simulink model "pitch_control_fuzzy"  (R2021b)
settings: Solver=VariableStepAuto  StartTime=0.0  StopTime=50  RelTol=1e-6
libraries: fuzblock x1
settings Model: Creator=Abner Souza  LastModifiedBy=Abner Souza

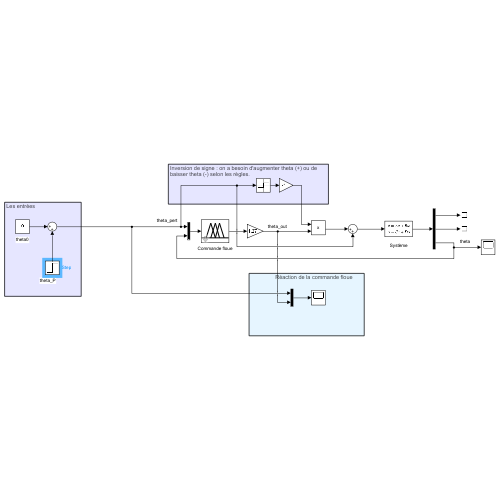
[thumbnail: Simulink's stored preview of the top-level diagram]
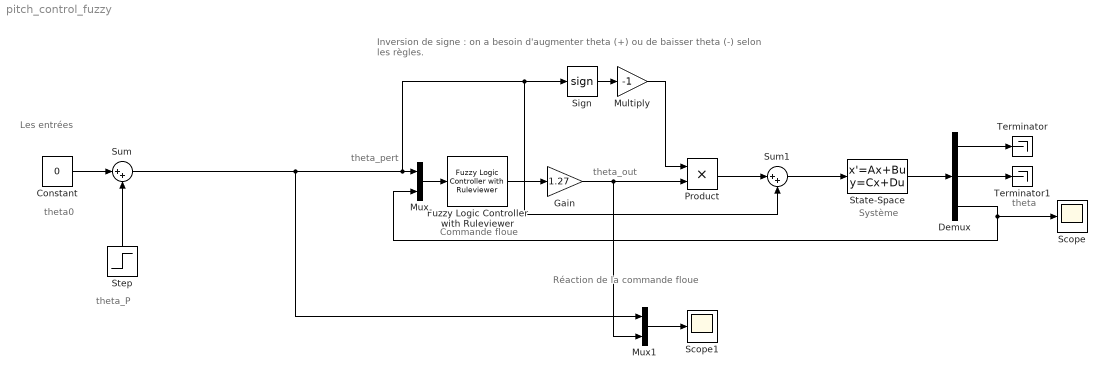
== system pitch_control_fuzzy ==
  note: Système
  note: Commande floue
  note: Inversion de signe : on a besoin d'augmenter theta (+) ou de
      | baisser theta (-) selon les règles.
  note: Réaction de la commande floue
  note: Les entrées
  note: theta_out
  note: theta_P
  note: theta0
  note: theta
  note: theta_pert
  Constant : Constant  Value=0
  Demux : Demux  Outputs=3
  Fuzzy Logic Controller with Ruleviewer : fuzblock/Fuzzy Logic  Controller  with Ruleviewer  fismatrix=rules_fuzzy  Ts=2
  Gain : Gain  Gain=1.27
  Multiply : Gain  Gain=-1
  Mux : Mux  Inputs=2
  Mux1 : Mux  Inputs=2
  Product : Product
  Scope : Scope
  Scope1 : Scope
  Sign : Signum
  State-Space : StateSpace  A=[-0.313 56.7 0; -0.0139 -0.426 0; 0 56.7 0]  B=[0.232; 0.0203; 0]  C=eye(3)  D=[0;0;0]  InitialCondition=0  ContinuousStateAttributes={'Angle_of_attack', 'Pitch_rate', 'Pitch_angle'}
  Step : Step  Time=0  After=0.2  SampleTime=0
  Sum : Sum  Inputs=|++
  Sum1 : Sum  Inputs=|++
  Terminator : Terminator
  Terminator1 : Terminator
  wires:
  Constant/1 -> Sum/1
  Step/1 -> Sum/2
  Sum/1 -> Mux1/1, Sign/1, Sum1/2, Mux/1
  Mux/1 -> Fuzzy Logic Controller with Ruleviewer/1
  State-Space/1 -> Demux/1
  Demux/1 -> Terminator/1
  Demux/2 -> Terminator1/1
  Demux/3 -> Mux/2, Scope/1
  Sign/1 -> Multiply/1
  Multiply/1 -> Product/1
  Product/1 -> Sum1/1
  Sum1/1 -> State-Space/1
  Mux1/1 -> Scope1/1
  Fuzzy Logic Controller with Ruleviewer/1 -> Gain/1
  Gain/1 -> Mux1/2, Product/2
